simulink model "read_write_1"  (Simulink 7.9)
settings: Solver=ode45  StartTime=0.0  StopTime=50000  RelTol=1e-3
libraries: xbsIndex_r4 x71, xps_library x1
settings Model: Creator=peter  LastModifiedBy=peter

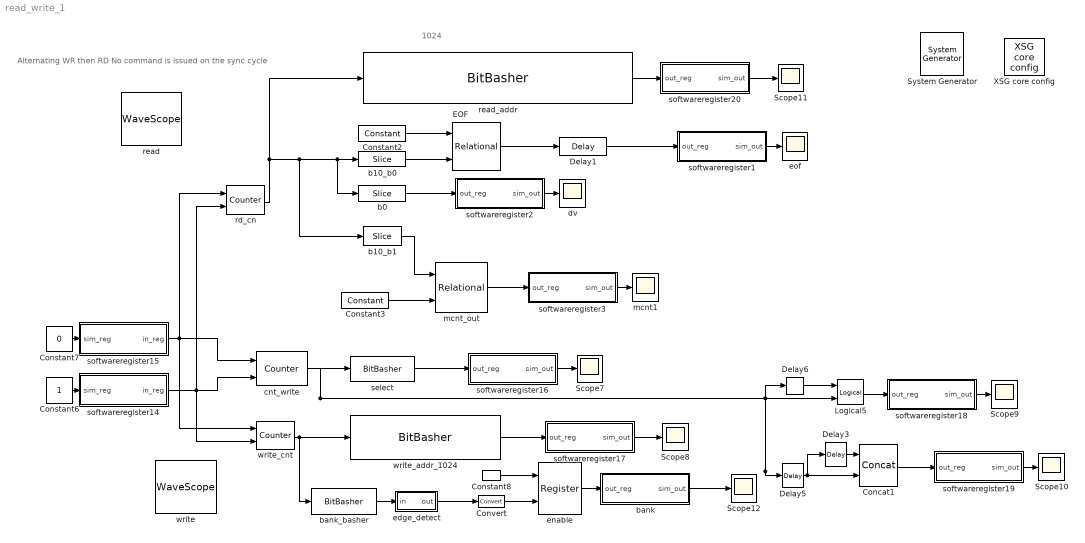
== system read_write_1 ==
  note: Alternating WR then RD
      | No command is issued
      | on the sync cycle
  note: 1024
  " System Generator" : xbsIndex_r4/ System Generator  Tag=genX  xilinxfamily=Kintex7  part=xc7k325t  speed=-3  package=fbg676  synthesis_tool=XST  clock_wrapper=Clock Enables  directory=./netlist  proj_type=Project Navigator  Synth_file=XST Defaults  Impl_file=ISE Defaults  testbench=off  simulink_period=1  sysclk_period=10  dcm_input_clock_period=10  incr_netlist=off  trim_vbits=Everywhere in SubSystem  dbl_ovrd=According to Block Masks  core_generation=According to Block Masks  run_coregen=off  deprecated_control=off  eval_field=0  block_type=sysgen
  Concat1 : xbsIndex_r4/Concat  num_inputs=2  dbl_ovrd=off  block_type=concat
      settings: block_version=10.1.3
  Constant2 : xbsIndex_r4/Constant  const=hex2dec('7FE')  gui_display_data_type=Fixed-point  arith_type=Unsigned  n_bits=11  bin_pt=0  preci_type=Single  exp_width=8  frac_width=24  explicit_period=on  period=1  equ=P=C  opselect=C  inp2=PCIN>>17  opr=+  inp1=P  carry=CIN  dbl_ovrd=off  block_type=constant
  Constant3 : xbsIndex_r4/Constant  const=hex2dec('7FE')  gui_display_data_type=Fixed-point  arith_type=Unsigned  n_bits=11  bin_pt=0  preci_type=Single  exp_width=8  frac_width=24  explicit_period=on  period=1  equ=P=C  opselect=C  inp2=PCIN>>17  opr=+  inp1=P  carry=CIN  dbl_ovrd=off  block_type=constant
  Constant6 : Constant
  Constant7 : Constant  Value=0
  Constant8 : xbsIndex_r4/Constant  const=1  gui_display_data_type=Boolean  arith_type=Boolean  n_bits=3  bin_pt=0  preci_type=Single  exp_width=8  frac_width=24  explicit_period=on  period=1  equ=P=C  opselect=C  inp2=PCIN>>17  opr=+  inp1=P  carry=CIN  dbl_ovrd=off  block_type=constant
  Convert : xbsIndex_r4/Convert  gui_display_data_type=Boolean  arith_type=Boolean  n_bits=16  bin_pt=14  float_type=Single  exp_bits=8  fraction_bits=24  quantization=Truncate  overflow=Wrap  en=off  latency=0  dbl_ovrd=off  pipeline=off  block_type=convert
  Delay1 : xbsIndex_r4/Delay  rst=off  infoeditControl=Selection of Reset will increase slice count due to use of real FFs and instead of SRLs  en=off  latency=1  dbl_ovrd=off  reg_retiming=off  block_type=delay
  Delay3 : xbsIndex_r4/Delay  rst=off  infoeditControl=Selection of Reset will increase slice count due to use of real FFs and instead of SRLs  en=off  latency=1  dbl_ovrd=off  reg_retiming=on  block_type=delay
      settings: xl_area=[0, 0, 0, 0, 0, 0, 0]
  Delay5 : xbsIndex_r4/Delay  rst=off  infoeditControl=Selection of Reset will increase slice count due to use of real FFs and instead of SRLs  en=off  latency=1  dbl_ovrd=off  reg_retiming=on  block_type=delay
      settings: xl_area=[0, 0, 0, 0, 0, 0, 0]
  Delay6 : xbsIndex_r4/Delay  rst=off  infoeditControl=Selection of Reset will increase slice count due to use of real FFs and instead of SRLs  en=off  latency=1  dbl_ovrd=off  reg_retiming=off  block_type=delay
      settings: xl_area=[0, 0, 0, 0, 0, 0, 0]
  EOF : xbsIndex_r4/Relational  mode=a=b  en=off  latency=1  dbl_ovrd=off  block_type=relational
  Logical5 : xbsIndex_r4/Logical  logical_function=XOR  inputs=2  en=off  latency=0  precision=Full  arith_type=Unsigned  n_bits=8  bin_pt=2  align_bp=on  dbl_ovrd=off  block_type=logical
      settings: xl_area=[0, 0, 0, 0, 0, 0, 0]
  Scope{7..12} (6 alike) : Scope
      Scope11 settings: ShowLegends=on  TimeRange=2500  YMin=0  YMax=8000  MaxDataPoints=1000000
      Scope12 settings: SaveName=ScopeData2
      Scope7 settings: YMin=-10  YMax=10  SaveName=ScopeData3
      Scope8 settings: ShowLegends=on  YMin=0  YMax=2050  SaveName=ScopeData4  MaxDataPoints=1000000
      Scope9 settings: SaveName=ScopeData5
  XSG core config : xps_library/XSG core config  Tag=xps:xsg  hw_sys=ROACH2:sx475t  clk_src=sys_clk  ROACH_clk_src=sys_clk  ROACH2_clk_src=sys_clk  clk_rate=100  sample_period=1  synthesis_tool=XST
  b0 : xbsIndex_r4/Slice  nbits=1  boolean_output=on  mode=Lower Bit Location + Width  bit1=0  base1=MSB of Input  bit0=0  base0=LSB of Input  dbl_ovrd=off  block_type=slice
  b10_b0 : xbsIndex_r4/Slice  nbits=11  boolean_output=off  mode=Lower Bit Location + Width  bit1=0  base1=MSB of Input  bit0=0  base0=LSB of Input  dbl_ovrd=off  block_type=slice
  b10_b1 : xbsIndex_r4/Slice  nbits=11  boolean_output=off  mode=Lower Bit Location + Width  bit1=0  base1=MSB of Input  bit0=0  base0=LSB of Input  dbl_ovrd=off  block_type=slice
  bank : Subsystem  Tag=xps:sw_reg  AncestorBlock=xps_library/software register  mask{numios=1, io_dir=To Processor, io_delay=0, sample_period=1, name1=reg, bitwidth1=1, arith_type1=Boolean, bin_pt1=0}
      mask prompts: numios "Num I/Os"; io_dir "I/O direction"; io_delay "I/O delay"; sample_period "Sample period"; name1 "Name"; bitwidth1 "Bitwidth"; arith_type1 "Type"; bin_pt1 "Binary pt"
      mask init:
      | swreg_init(gcb);
      mask StyleString: edit,popup(To Processor|From Processor),edit,edit,edit,edit,popup(Unsigned|Signed  (2's comp)|Boolean),edit
      mask CallbackString:
      | t = timer('StartDelay', 0.1); t.TimerFcn = {@swreg_cb, gcb}; start(t);|a = get_param(gcb, 'MaskEnables');
      | if strcmp(get_param(gcb, 'io_dir'), 'To Processor'),
      | a(4) = {'off'};
      | else
      | a(4) = {'on'};
      | end
      | set_param(gcb, 'MaskEnables', a);
      | |||||a = get_param(gcb, 'MaskEnables');
      | if strcmp(get_param(gcb, 'arith_type1'), 'Boolean'),
      | set_param(gcb, 'bitwidth1', '1');
      | set_param(gcb, 'bin_pt1', '0');
      | a(6) = {'off'};
      | a(8) = {'off'};
      | else
      | a(6) = {'on'};
      | a(8) = {'on'};
      | end
      | set_param(gcb, 'MaskEnables', a);
      | |
      mask TabNameString: Setup,Setup,Setup,Setup,IO1,IO1,IO1,IO1
  bank_basher : xbsIndex_r4/BitBasher  bitexpr=b={a[14]}  display_expr=on  sr_1=1  arith_type1=Unsigned  bin_pt1=0  sr_2=2  arith_type2=Unsigned  bin_pt2=0  sr_3=3  arith_type3=Unsigned  bin_pt3=0  sr_4=4  arith_type4=Unsigned  bin_pt4=0  dbl_ovrd=off  block_type=bitbasher
  cnt_write : xbsIndex_r4/Counter  cnt_type=Free Running  cnt_to=Inf  operation=Up  start_count=0  cnt_by_val=1  arith_type=Unsigned  n_bits=14  bin_pt=0  load_pin=off  rst=on  en=on  explicit_period=on  period=1  dbl_ovrd=off  use_behavioral_HDL=off  implementation=Fabric  use_rpm=off  block_type=counter
  dv : Scope
      settings: SaveName=ScopeData7
  edge_detect : Subsystem  AncestorBlock=casper_library_misc/edge_detect  mask(edge_detect){edge=Rising, polarity=Active High, x_in=[0 0.08 0.08 0.16 0.16 0.24 0.24 0.32 0.32 0.4], y_in=[-1 -1  1  1  1  1  1  1  1  1], x_out=[0.6 0.68 0.68 0.76 0.76 0.84 0.84 0.92 0.92 1], y_out=[-1 -1  1  1 -1 -1 -1 -1 -1 -1]}
      mask prompts: edge "Edge Type"; polarity "Output Polarity"; x_in "Input X Positions"; y_in "Input Y Positions"; x_out "Output X Positions"; y_out "Output Y Positions"
      mask help: Output is active for one-cycle after each edge of the specified type (i.e. rising, falling or both).
      mask init:
      | edge_detect_init(gcb,...
      |     'edge',edge,...
      |     'polarity',polarity,...
      |     'x_in',x_in,...
      |     'x_out',x_out,...
      |     'y_in',y_in,...
      |     'y_out',y_out);
      | 
      | x_in_num=str2num(getfield(getfield(get_param(gcb,'UserData'),'parameters'),'x_in'));
      | x_out_num=str2num(getfield(getfield(get_param(gcb,'UserData'),'parameters'),'x_out'));
      | y_in_num=str2num(getfield(getfield(get_param(gcb,'UserData'),'parameters'),'y_in'));
      | y_out_num=str2num(getfield(getfield(get_param(gcb,'UserData'),'parameters'),'y_out'));
      settings: AttributesFormatString=|
      | rising edges
      | active high
      mask Help: Output is active for one-cycle after each edge of the specified type (i.e. rising, falling, or both).  Latency is zero.
      mask StyleString: popup(Rising|Falling|Both),popup(Active High|Active Low),edit,edit,edit,edit
      mask Display:
      | plot(x_in_num,0.5+y_in_num*0.2);
      | plot(x_out_num,0.5+y_out_num*0.2);
  enable : xbsIndex_r4/Register  init=0  rst=off  en=on  dbl_ovrd=off  block_type=register
  eof : Scope
      settings: SaveName=ScopeData6
  mcnt1 : Scope
      settings: SaveName=ScopeData8
  mcnt_out : xbsIndex_r4/Relational  mode=a=b  en=off  latency=0  dbl_ovrd=off  block_type=relational
  rd_cn : xbsIndex_r4/Counter  cnt_type=Free Running  cnt_to=Inf  operation=Up  start_count=hex2dec('7FFE')  cnt_by_val=1  arith_type=Unsigned  n_bits=15  bin_pt=0  load_pin=off  rst=on  en=on  explicit_period=on  period=1  dbl_ovrd=off  use_behavioral_HDL=on  implementation=Fabric  use_rpm=off  block_type=counter
  read : xbsIndex_r4/WaveScope  block_type=wavescope
  read_addr : xbsIndex_r4/BitBasher  bitexpr=b={a[14],a[13:11],a[2],a[10:3],a[1]}  display_expr=on  sr_1=1  arith_type1=Unsigned  bin_pt1=0  sr_2=2  arith_type2=Unsigned  bin_pt2=0  sr_3=3  arith_type3=Unsigned  bin_pt3=0  sr_4=4  arith_type4=Unsigned  bin_pt4=0  dbl_ovrd=off  block_type=bitbasher
  select : xbsIndex_r4/BitBasher  bitexpr=b={a[8:7]}  display_expr=on  sr_1=1  arith_type1=Unsigned  bin_pt1=0  sr_2=2  arith_type2=Unsigned  bin_pt2=0  sr_3=3  arith_type3=Unsigned  bin_pt3=0  sr_4=4  arith_type4=Unsigned  bin_pt4=0  dbl_ovrd=off  block_type=bitbasher
  softwareregister1 : Subsystem  Tag=xps:sw_reg  AncestorBlock=xps_library/software register  mask{numios=1, io_dir=To Processor, io_delay=0, sample_period=1, name1=reg, bitwidth1=32, arith_type1=Unsigned, bin_pt1=0}
      mask prompts: numios "Num I/Os"; io_dir "I/O direction"; io_delay "I/O delay"; sample_period "Sample period"; name1 "Name"; bitwidth1 "Bitwidth"; arith_type1 "Type"; bin_pt1 "Binary pt"
      mask init:
      | swreg_init(gcb);
      mask StyleString: edit,popup(To Processor|From Processor),edit,edit,edit,edit,popup(Unsigned|Signed  (2's comp)|Boolean),edit
      mask CallbackString:
      | t = timer('StartDelay', 0.1); t.TimerFcn = {@swreg_cb, gcb}; start(t);|a = get_param(gcb, 'MaskEnables');
      | if strcmp(get_param(gcb, 'io_dir'), 'To Processor'),
      | a(4) = {'off'};
      | else
      | a(4) = {'on'};
      | end
      | set_param(gcb, 'MaskEnables', a);
      | |||||a = get_param(gcb, 'MaskEnables');
      | if strcmp(get_param(gcb, 'arith_type1'), 'Boolean'),
      | set_param(gcb, 'bitwidth1', '1');
      | set_param(gcb, 'bin_pt1', '0');
      | a(6) = {'off'};
      | a(8) = {'off'};
      | else
      | a(6) = {'on'};
      | a(8) = {'on'};
      | end
      | set_param(gcb, 'MaskEnables', a);
      | |
      mask TabNameString: Setup,Setup,Setup,Setup,IO1,IO1,IO1,IO1
  softwareregister14 : Subsystem  Tag=xps:sw_reg  AncestorBlock=xps_library/software register  mask{numios=1, io_dir=From Processor, io_delay=0, sample_period=1, name1=reg, bitwidth1=1, arith_type1=Boolean, bin_pt1=0}
      mask prompts: numios "Num I/Os"; io_dir "I/O direction"; io_delay "I/O delay"; sample_period "Sample period"; name1 "Name"; bitwidth1 "Bitwidth"; arith_type1 "Type"; bin_pt1 "Binary pt"
      mask init:
      | swreg_init(gcb);
      mask StyleString: edit,popup(To Processor|From Processor),edit,edit,edit,edit,popup(Unsigned|Signed  (2's comp)|Boolean),edit
      mask CallbackString:
      | t = timer('StartDelay', 0.1); t.TimerFcn = {@swreg_cb, gcb}; start(t);|a = get_param(gcb, 'MaskEnables');
      | if strcmp(get_param(gcb, 'io_dir'), 'To Processor'),
      | a(4) = {'off'};
      | else
      | a(4) = {'on'};
      | end
      | set_param(gcb, 'MaskEnables', a);
      | |||||a = get_param(gcb, 'MaskEnables');
      | if strcmp(get_param(gcb, 'arith_type1'), 'Boolean'),
      | set_param(gcb, 'bitwidth1', '1');
      | set_param(gcb, 'bin_pt1', '0');
      | a(6) = {'off'};
      | a(8) = {'off'};
      | else
      | a(6) = {'on'};
      | a(8) = {'on'};
      | end
      | set_param(gcb, 'MaskEnables', a);
      | |
      mask TabNameString: Setup,Setup,Setup,Setup,IO1,IO1,IO1,IO1
  softwareregister15 : Subsystem  Tag=xps:sw_reg  AncestorBlock=xps_library/software register  mask{numios=1, io_dir=From Processor, io_delay=0, sample_period=1, name1=reg, bitwidth1=1, arith_type1=Boolean, bin_pt1=0}
      mask prompts: numios "Num I/Os"; io_dir "I/O direction"; io_delay "I/O delay"; sample_period "Sample period"; name1 "Name"; bitwidth1 "Bitwidth"; arith_type1 "Type"; bin_pt1 "Binary pt"
      mask init:
      | swreg_init(gcb);
      mask StyleString: edit,popup(To Processor|From Processor),edit,edit,edit,edit,popup(Unsigned|Signed  (2's comp)|Boolean),edit
      mask CallbackString:
      | t = timer('StartDelay', 0.1); t.TimerFcn = {@swreg_cb, gcb}; start(t);|a = get_param(gcb, 'MaskEnables');
      | if strcmp(get_param(gcb, 'io_dir'), 'To Processor'),
      | a(4) = {'off'};
      | else
      | a(4) = {'on'};
      | end
      | set_param(gcb, 'MaskEnables', a);
      | |||||a = get_param(gcb, 'MaskEnables');
      | if strcmp(get_param(gcb, 'arith_type1'), 'Boolean'),
      | set_param(gcb, 'bitwidth1', '1');
      | set_param(gcb, 'bin_pt1', '0');
      | a(6) = {'off'};
      | a(8) = {'off'};
      | else
      | a(6) = {'on'};
      | a(8) = {'on'};
      | end
      | set_param(gcb, 'MaskEnables', a);
      | |
      mask TabNameString: Setup,Setup,Setup,Setup,IO1,IO1,IO1,IO1
  softwareregister16 : Subsystem  Tag=xps:sw_reg  AncestorBlock=xps_library/software register  mask{numios=1, io_dir=To Processor, io_delay=0, sample_period=1, name1=reg, bitwidth1=32, arith_type1=Unsigned, bin_pt1=0}
      mask prompts: numios "Num I/Os"; io_dir "I/O direction"; io_delay "I/O delay"; sample_period "Sample period"; name1 "Name"; bitwidth1 "Bitwidth"; arith_type1 "Type"; bin_pt1 "Binary pt"
      mask init:
      | swreg_init(gcb);
      mask StyleString: edit,popup(To Processor|From Processor),edit,edit,edit,edit,popup(Unsigned|Signed  (2's comp)|Boolean),edit
      mask CallbackString:
      | t = timer('StartDelay', 0.1); t.TimerFcn = {@swreg_cb, gcb}; start(t);|a = get_param(gcb, 'MaskEnables');
      | if strcmp(get_param(gcb, 'io_dir'), 'To Processor'),
      | a(4) = {'off'};
      | else
      | a(4) = {'on'};
      | end
      | set_param(gcb, 'MaskEnables', a);
      | |||||a = get_param(gcb, 'MaskEnables');
      | if strcmp(get_param(gcb, 'arith_type1'), 'Boolean'),
      | set_param(gcb, 'bitwidth1', '1');
      | set_param(gcb, 'bin_pt1', '0');
      | a(6) = {'off'};
      | a(8) = {'off'};
      | else
      | a(6) = {'on'};
      | a(8) = {'on'};
      | end
      | set_param(gcb, 'MaskEnables', a);
      | |
      mask TabNameString: Setup,Setup,Setup,Setup,IO1,IO1,IO1,IO1
  softwareregister17 : Subsystem  Tag=xps:sw_reg  AncestorBlock=xps_library/software register  mask{numios=1, io_dir=To Processor, io_delay=0, sample_period=1, name1=reg, bitwidth1=14, arith_type1=Unsigned, bin_pt1=0}
      mask prompts: numios "Num I/Os"; io_dir "I/O direction"; io_delay "I/O delay"; sample_period "Sample period"; name1 "Name"; bitwidth1 "Bitwidth"; arith_type1 "Type"; bin_pt1 "Binary pt"
      mask init:
      | swreg_init(gcb);
      mask StyleString: edit,popup(To Processor|From Processor),edit,edit,edit,edit,popup(Unsigned|Signed  (2's comp)|Boolean),edit
      mask CallbackString:
      | t = timer('StartDelay', 0.1); t.TimerFcn = {@swreg_cb, gcb}; start(t);|a = get_param(gcb, 'MaskEnables');
      | if strcmp(get_param(gcb, 'io_dir'), 'To Processor'),
      | a(4) = {'off'};
      | else
      | a(4) = {'on'};
      | end
      | set_param(gcb, 'MaskEnables', a);
      | |||||a = get_param(gcb, 'MaskEnables');
      | if strcmp(get_param(gcb, 'arith_type1'), 'Boolean'),
      | set_param(gcb, 'bitwidth1', '1');
      | set_param(gcb, 'bin_pt1', '0');
      | a(6) = {'off'};
      | a(8) = {'off'};
      | else
      | a(6) = {'on'};
      | a(8) = {'on'};
      | end
      | set_param(gcb, 'MaskEnables', a);
      | |
      mask TabNameString: Setup,Setup,Setup,Setup,IO1,IO1,IO1,IO1
  softwareregister18 : Subsystem  Tag=xps:sw_reg  AncestorBlock=xps_library/software register  mask{numios=1, io_dir=To Processor, io_delay=0, sample_period=1, name1=reg, bitwidth1=32, arith_type1=Unsigned, bin_pt1=0}
      mask prompts: numios "Num I/Os"; io_dir "I/O direction"; io_delay "I/O delay"; sample_period "Sample period"; name1 "Name"; bitwidth1 "Bitwidth"; arith_type1 "Type"; bin_pt1 "Binary pt"
      mask init:
      | swreg_init(gcb);
      mask StyleString: edit,popup(To Processor|From Processor),edit,edit,edit,edit,popup(Unsigned|Signed  (2's comp)|Boolean),edit
      mask CallbackString:
      | t = timer('StartDelay', 0.1); t.TimerFcn = {@swreg_cb, gcb}; start(t);|a = get_param(gcb, 'MaskEnables');
      | if strcmp(get_param(gcb, 'io_dir'), 'To Processor'),
      | a(4) = {'off'};
      | else
      | a(4) = {'on'};
      | end
      | set_param(gcb, 'MaskEnables', a);
      | |||||a = get_param(gcb, 'MaskEnables');
      | if strcmp(get_param(gcb, 'arith_type1'), 'Boolean'),
      | set_param(gcb, 'bitwidth1', '1');
      | set_param(gcb, 'bin_pt1', '0');
      | a(6) = {'off'};
      | a(8) = {'off'};
      | else
      | a(6) = {'on'};
      | a(8) = {'on'};
      | end
      | set_param(gcb, 'MaskEnables', a);
      | |
      mask TabNameString: Setup,Setup,Setup,Setup,IO1,IO1,IO1,IO1
  softwareregister19 : Subsystem  Tag=xps:sw_reg  AncestorBlock=xps_library/software register  mask{numios=1, io_dir=To Processor, io_delay=0, sample_period=1, name1=reg, bitwidth1=32, arith_type1=Unsigned, bin_pt1=0}
      mask prompts: numios "Num I/Os"; io_dir "I/O direction"; io_delay "I/O delay"; sample_period "Sample period"; name1 "Name"; bitwidth1 "Bitwidth"; arith_type1 "Type"; bin_pt1 "Binary pt"
      mask init:
      | swreg_init(gcb);
      mask StyleString: edit,popup(To Processor|From Processor),edit,edit,edit,edit,popup(Unsigned|Signed  (2's comp)|Boolean),edit
      mask CallbackString:
      | t = timer('StartDelay', 0.1); t.TimerFcn = {@swreg_cb, gcb}; start(t);|a = get_param(gcb, 'MaskEnables');
      | if strcmp(get_param(gcb, 'io_dir'), 'To Processor'),
      | a(4) = {'off'};
      | else
      | a(4) = {'on'};
      | end
      | set_param(gcb, 'MaskEnables', a);
      | |||||a = get_param(gcb, 'MaskEnables');
      | if strcmp(get_param(gcb, 'arith_type1'), 'Boolean'),
      | set_param(gcb, 'bitwidth1', '1');
      | set_param(gcb, 'bin_pt1', '0');
      | a(6) = {'off'};
      | a(8) = {'off'};
      | else
      | a(6) = {'on'};
      | a(8) = {'on'};
      | end
      | set_param(gcb, 'MaskEnables', a);
      | |
      mask TabNameString: Setup,Setup,Setup,Setup,IO1,IO1,IO1,IO1
  softwareregister2 : Subsystem  Tag=xps:sw_reg  AncestorBlock=xps_library/software register  mask{numios=1, io_dir=To Processor, io_delay=0, sample_period=1, name1=reg, bitwidth1=32, arith_type1=Unsigned, bin_pt1=0}
      mask prompts: numios "Num I/Os"; io_dir "I/O direction"; io_delay "I/O delay"; sample_period "Sample period"; name1 "Name"; bitwidth1 "Bitwidth"; arith_type1 "Type"; bin_pt1 "Binary pt"
      mask init:
      | swreg_init(gcb);
      mask StyleString: edit,popup(To Processor|From Processor),edit,edit,edit,edit,popup(Unsigned|Signed  (2's comp)|Boolean),edit
      mask CallbackString:
      | t = timer('StartDelay', 0.1); t.TimerFcn = {@swreg_cb, gcb}; start(t);|a = get_param(gcb, 'MaskEnables');
      | if strcmp(get_param(gcb, 'io_dir'), 'To Processor'),
      | a(4) = {'off'};
      | else
      | a(4) = {'on'};
      | end
      | set_param(gcb, 'MaskEnables', a);
      | |||||a = get_param(gcb, 'MaskEnables');
      | if strcmp(get_param(gcb, 'arith_type1'), 'Boolean'),
      | set_param(gcb, 'bitwidth1', '1');
      | set_param(gcb, 'bin_pt1', '0');
      | a(6) = {'off'};
      | a(8) = {'off'};
      | else
      | a(6) = {'on'};
      | a(8) = {'on'};
      | end
      | set_param(gcb, 'MaskEnables', a);
      | |
      mask TabNameString: Setup,Setup,Setup,Setup,IO1,IO1,IO1,IO1
  softwareregister20 : Subsystem  Tag=xps:sw_reg  AncestorBlock=xps_library/software register  mask{numios=1, io_dir=To Processor, io_delay=0, sample_period=1, name1=reg, bitwidth1=15, arith_type1=Unsigned, bin_pt1=0}
      mask prompts: numios "Num I/Os"; io_dir "I/O direction"; io_delay "I/O delay"; sample_period "Sample period"; name1 "Name"; bitwidth1 "Bitwidth"; arith_type1 "Type"; bin_pt1 "Binary pt"
      mask init:
      | swreg_init(gcb);
      mask StyleString: edit,popup(To Processor|From Processor),edit,edit,edit,edit,popup(Unsigned|Signed  (2's comp)|Boolean),edit
      mask CallbackString:
      | t = timer('StartDelay', 0.1); t.TimerFcn = {@swreg_cb, gcb}; start(t);|a = get_param(gcb, 'MaskEnables');
      | if strcmp(get_param(gcb, 'io_dir'), 'To Processor'),
      | a(4) = {'off'};
      | else
      | a(4) = {'on'};
      | end
      | set_param(gcb, 'MaskEnables', a);
      | |||||a = get_param(gcb, 'MaskEnables');
      | if strcmp(get_param(gcb, 'arith_type1'), 'Boolean'),
      | set_param(gcb, 'bitwidth1', '1');
      | set_param(gcb, 'bin_pt1', '0');
      | a(6) = {'off'};
      | a(8) = {'off'};
      | else
      | a(6) = {'on'};
      | a(8) = {'on'};
      | end
      | set_param(gcb, 'MaskEnables', a);
      | |
      mask TabNameString: Setup,Setup,Setup,Setup,IO1,IO1,IO1,IO1
  softwareregister3 : Subsystem  Tag=xps:sw_reg  AncestorBlock=xps_library/software register  mask{numios=1, io_dir=To Processor, io_delay=0, sample_period=1, name1=reg, bitwidth1=32, arith_type1=Unsigned, bin_pt1=0}
      mask prompts: numios "Num I/Os"; io_dir "I/O direction"; io_delay "I/O delay"; sample_period "Sample period"; name1 "Name"; bitwidth1 "Bitwidth"; arith_type1 "Type"; bin_pt1 "Binary pt"
      mask init:
      | swreg_init(gcb);
      mask StyleString: edit,popup(To Processor|From Processor),edit,edit,edit,edit,popup(Unsigned|Signed  (2's comp)|Boolean),edit
      mask CallbackString:
      | t = timer('StartDelay', 0.1); t.TimerFcn = {@swreg_cb, gcb}; start(t);|a = get_param(gcb, 'MaskEnables');
      | if strcmp(get_param(gcb, 'io_dir'), 'To Processor'),
      | a(4) = {'off'};
      | else
      | a(4) = {'on'};
      | end
      | set_param(gcb, 'MaskEnables', a);
      | |||||a = get_param(gcb, 'MaskEnables');
      | if strcmp(get_param(gcb, 'arith_type1'), 'Boolean'),
      | set_param(gcb, 'bitwidth1', '1');
      | set_param(gcb, 'bin_pt1', '0');
      | a(6) = {'off'};
      | a(8) = {'off'};
      | else
      | a(6) = {'on'};
      | a(8) = {'on'};
      | end
      | set_param(gcb, 'MaskEnables', a);
      | |
      mask TabNameString: Setup,Setup,Setup,Setup,IO1,IO1,IO1,IO1
  write : xbsIndex_r4/WaveScope  block_type=wavescope
  write_addr_1024 : xbsIndex_r4/BitBasher  bitexpr=b={a[14:10],a[7:0]}  display_expr=on  sr_1=1  arith_type1=Unsigned  bin_pt1=0  sr_2=2  arith_type2=Unsigned  bin_pt2=0  sr_3=3  arith_type3=Unsigned  bin_pt3=0  sr_4=4  arith_type4=Unsigned  bin_pt4=0  dbl_ovrd=off  block_type=bitbasher
  write_cnt : xbsIndex_r4/Counter  cnt_type=Free Running  cnt_to=Inf  operation=Up  start_count=0  cnt_by_val=1  arith_type=Unsigned  n_bits=15  bin_pt=0  load_pin=off  rst=on  en=on  explicit_period=on  period=1  dbl_ovrd=off  use_behavioral_HDL=off  implementation=Fabric  use_rpm=off  block_type=counter
  wires:
  Constant6/1 -> softwareregister14/1(sim_reg)
  Constant7/1 -> softwareregister15/1(sim_reg)
  softwareregister15/1(in_reg) -> cnt_write/1, write_cnt/1, rd_cn/1
  softwareregister14/1(in_reg) -> cnt_write/2, write_cnt/2, rd_cn/2
  cnt_write/1 -> Delay6/1, Logical5/2, Delay5/1, select/1
  softwareregister16/1(sim_out) -> Scope7/1
  write_cnt/1 -> write_addr_1024/1, bank_basher/1
  softwareregister17/1(sim_out) -> Scope8/1
  write_addr_1024/1 -> softwareregister17/1(out_reg)
  Delay6/1 -> Logical5/1
  Logical5/1 -> softwareregister18/1(out_reg)
  softwareregister18/1(sim_out) -> Scope9/1
  Delay3/1 -> Concat1/1
  Delay5/1 -> Concat1/2, Delay3/1
  softwareregister19/1(sim_out) -> Scope10/1
  Concat1/1 -> softwareregister19/1(out_reg)
  softwareregister20/1(sim_out) -> Scope11/1
  read_addr/1 -> softwareregister20/1(out_reg)
  rd_cn/1 -> read_addr/1, b10_b0/1, b0/1, b10_b1/1
  select/1 -> softwareregister16/1(out_reg)
  bank/1(sim_out) -> Scope12/1
  bank_basher/1 -> edge_detect/1(in)
  Constant8/1 -> enable/1
  edge_detect/1(out) -> Convert/1
  enable/1 -> bank/1(out_reg)
  Convert/1 -> enable/2
  Constant2/1 -> EOF/1
  b10_b0/1 -> EOF/2
  EOF/1 -> Delay1/1
  softwareregister1/1(sim_out) -> eof/1
  Delay1/1 -> softwareregister1/1(out_reg)
  softwareregister2/1(sim_out) -> dv/1
  b0/1 -> softwareregister2/1(out_reg)
  softwareregister3/1(sim_out) -> mcnt1/1
  Constant3/1 -> mcnt_out/2
  mcnt_out/1 -> softwareregister3/1(out_reg)
  b10_b1/1 -> mcnt_out/1

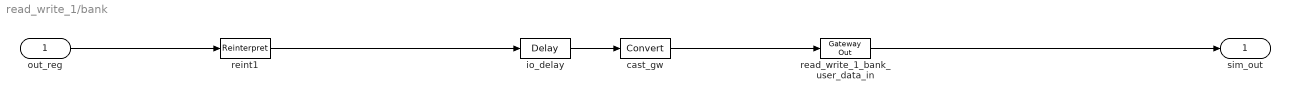
== system read_write_1/bank ==
  out_reg : Inport
  cast_gw : xbsIndex_r4/Convert  gui_display_data_type=Fixed-point  arith_type=Unsigned  n_bits=32  bin_pt=0  float_type=Single  exp_bits=8  fraction_bits=24  quantization=Truncate  overflow=Wrap  en=off  latency=0  dbl_ovrd=off  pipeline=off  block_type=convert
  io_delay : xbsIndex_r4/Delay  rst=off  infoeditControl=Selection of Reset will increase slice count due to use of real FFs and instead of SRLs  en=off  latency=0  dbl_ovrd=off  reg_retiming=on  block_type=delay
  read_write_1_bank_user_data_in : xbsIndex_r4/Gateway Out  inherit_from_input=off  hdl_port=on  timing_constraint=None  locs_specified=off  LOCs={}  UseAsDAC=off  DACChannel='1'  block_type=gatewayout
  reint1 : xbsIndex_r4/Reinterpret  force_arith_type=on  arith_type=Unsigned  force_bin_pt=on  bin_pt=0  block_type=reinterpret
  sim_out : Outport
  wires:
  io_delay/1 -> cast_gw/1
  cast_gw/1 -> read_write_1_bank_user_data_in/1
  read_write_1_bank_user_data_in/1 -> sim_out/1
  out_reg/1 -> reint1/1
  reint1/1 -> io_delay/1

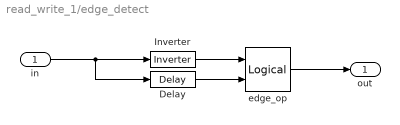
== system read_write_1/edge_detect ==
  in : Inport
  Delay : xbsIndex_r4/Delay  rst=off  infoeditControl=Selection of Reset will increase slice count due to use of real FFs and instead of SRLs  en=off  latency=1  dbl_ovrd=off  reg_retiming=off  block_type=delay
      settings: xl_area=[0, 0, 0, 0, 0, 0, 0]
  Inverter : xbsIndex_r4/Inverter  en=off  latency=0  dbl_ovrd=off  block_type=inv
      settings: xl_area=[0, 0, 0, 0, 0, 0, 0]
  edge_op : xbsIndex_r4/Logical  logical_function=NOR  inputs=2  en=off  latency=0  precision=Full  arith_type=Unsigned  n_bits=8  bin_pt=2  align_bp=on  dbl_ovrd=off  block_type=logical
      settings: xl_area=[0, 0, 0, 0, 0, 0, 0]
  out : Outport
  wires:
  Inverter/1 -> edge_op/1
  edge_op/1 -> out/1
  in/1 -> Inverter/1, Delay/1
  Delay/1 -> edge_op/2

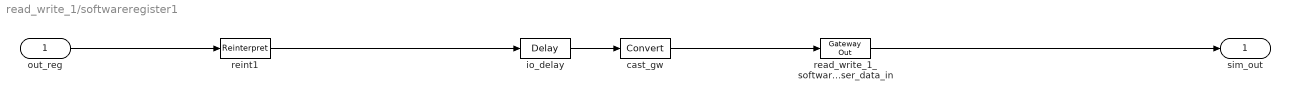
== system read_write_1/softwareregister1 ==
  out_reg : Inport
  cast_gw : xbsIndex_r4/Convert  gui_display_data_type=Fixed-point  arith_type=Unsigned  n_bits=32  bin_pt=0  float_type=Single  exp_bits=8  fraction_bits=24  quantization=Truncate  overflow=Wrap  en=off  latency=0  dbl_ovrd=off  pipeline=off  block_type=convert
  io_delay : xbsIndex_r4/Delay  rst=off  infoeditControl=Selection of Reset will increase slice count due to use of real FFs and instead of SRLs  en=off  latency=0  dbl_ovrd=off  reg_retiming=on  block_type=delay
  read_write_1_softwareregister1_user_data_in : xbsIndex_r4/Gateway Out  inherit_from_input=off  hdl_port=on  timing_constraint=None  locs_specified=off  LOCs={}  UseAsDAC=off  DACChannel='1'  block_type=gatewayout
  reint1 : xbsIndex_r4/Reinterpret  force_arith_type=on  arith_type=Unsigned  force_bin_pt=on  bin_pt=0  block_type=reinterpret
  sim_out : Outport
  wires:
  io_delay/1 -> cast_gw/1
  cast_gw/1 -> read_write_1_softwareregister1_user_data_in/1
  read_write_1_softwareregister1_user_data_in/1 -> sim_out/1
  out_reg/1 -> reint1/1
  reint1/1 -> io_delay/1

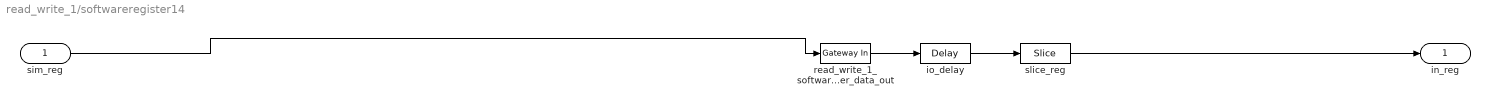
== system read_write_1/softwareregister14 ==
  sim_reg : Inport
  io_delay : xbsIndex_r4/Delay  rst=off  infoeditControl=Selection of Reset will increase slice count due to use of real FFs and instead of SRLs  en=off  latency=0  dbl_ovrd=off  reg_retiming=on  block_type=delay
  read_write_1_softwareregister14_user_data_out : xbsIndex_r4/Gateway In  gui_display_data_type=Fixed-point  arith_type=Unsigned  n_bits=32  bin_pt=0  preci_type=Single  exp_width=8  frac_width=24  quantization="Round  (unbiased: +/- Inf)"  overflow=Saturate  period=1  dbl_ovrd=off  timing_constraint=None  locs_specified=off  LOCs={}  UseAsADC=off  ADCChannel='1'  inherit_from_input=off  hdl_port=on  block_type=gatewayin
  slice_reg : xbsIndex_r4/Slice  nbits=1  boolean_output=on  mode=Lower Bit Location + Width  bit1=0  base1=MSB of Input  bit0=0  base0=LSB of Input  dbl_ovrd=off  block_type=slice
  in_reg : Outport
  wires:
  read_write_1_softwareregister14_user_data_out/1 -> io_delay/1
  sim_reg/1 -> read_write_1_softwareregister14_user_data_out/1
  io_delay/1 -> slice_reg/1
  slice_reg/1 -> in_reg/1

== system read_write_1/softwareregister15 ==
  sim_reg : Inport
  io_delay : xbsIndex_r4/Delay  rst=off  infoeditControl=Selection of Reset will increase slice count due to use of real FFs and instead of SRLs  en=off  latency=0  dbl_ovrd=off  reg_retiming=on  block_type=delay
  read_write_1_softwareregister15_user_data_out : xbsIndex_r4/Gateway In  gui_display_data_type=Fixed-point  arith_type=Unsigned  n_bits=32  bin_pt=0  preci_type=Single  exp_width=8  frac_width=24  quantization="Round  (unbiased: +/- Inf)"  overflow=Saturate  period=1  dbl_ovrd=off  timing_constraint=None  locs_specified=off  LOCs={}  UseAsADC=off  ADCChannel='1'  inherit_from_input=off  hdl_port=on  block_type=gatewayin
  slice_reg : xbsIndex_r4/Slice  nbits=1  boolean_output=on  mode=Lower Bit Location + Width  bit1=0  base1=MSB of Input  bit0=0  base0=LSB of Input  dbl_ovrd=off  block_type=slice
  in_reg : Outport
  wires:
  read_write_1_softwareregister15_user_data_out/1 -> io_delay/1
  sim_reg/1 -> read_write_1_softwareregister15_user_data_out/1
  io_delay/1 -> slice_reg/1
  slice_reg/1 -> in_reg/1

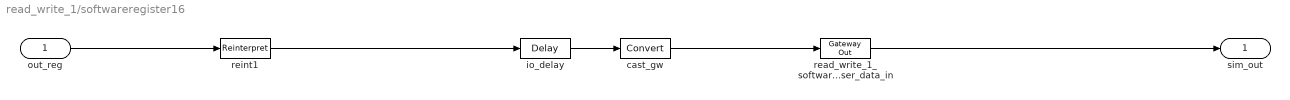
== system read_write_1/softwareregister16 ==
  out_reg : Inport
  cast_gw : xbsIndex_r4/Convert  gui_display_data_type=Fixed-point  arith_type=Unsigned  n_bits=32  bin_pt=0  float_type=Single  exp_bits=8  fraction_bits=24  quantization=Truncate  overflow=Wrap  en=off  latency=0  dbl_ovrd=off  pipeline=off  block_type=convert
  io_delay : xbsIndex_r4/Delay  rst=off  infoeditControl=Selection of Reset will increase slice count due to use of real FFs and instead of SRLs  en=off  latency=0  dbl_ovrd=off  reg_retiming=on  block_type=delay
  read_write_1_softwareregister16_user_data_in : xbsIndex_r4/Gateway Out  inherit_from_input=off  hdl_port=on  timing_constraint=None  locs_specified=off  LOCs={}  UseAsDAC=off  DACChannel='1'  block_type=gatewayout
  reint1 : xbsIndex_r4/Reinterpret  force_arith_type=on  arith_type=Unsigned  force_bin_pt=on  bin_pt=0  block_type=reinterpret
  sim_out : Outport
  wires:
  io_delay/1 -> cast_gw/1
  cast_gw/1 -> read_write_1_softwareregister16_user_data_in/1
  read_write_1_softwareregister16_user_data_in/1 -> sim_out/1
  out_reg/1 -> reint1/1
  reint1/1 -> io_delay/1

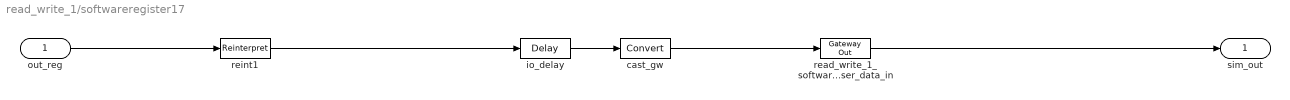
== system read_write_1/softwareregister17 ==
  out_reg : Inport
  cast_gw : xbsIndex_r4/Convert  gui_display_data_type=Fixed-point  arith_type=Unsigned  n_bits=32  bin_pt=0  float_type=Single  exp_bits=8  fraction_bits=24  quantization=Truncate  overflow=Wrap  en=off  latency=0  dbl_ovrd=off  pipeline=off  block_type=convert
  io_delay : xbsIndex_r4/Delay  rst=off  infoeditControl=Selection of Reset will increase slice count due to use of real FFs and instead of SRLs  en=off  latency=0  dbl_ovrd=off  reg_retiming=on  block_type=delay
  read_write_1_softwareregister17_user_data_in : xbsIndex_r4/Gateway Out  inherit_from_input=off  hdl_port=on  timing_constraint=None  locs_specified=off  LOCs={}  UseAsDAC=off  DACChannel='1'  block_type=gatewayout
  reint1 : xbsIndex_r4/Reinterpret  force_arith_type=on  arith_type=Unsigned  force_bin_pt=on  bin_pt=0  block_type=reinterpret
  sim_out : Outport
  wires:
  io_delay/1 -> cast_gw/1
  cast_gw/1 -> read_write_1_softwareregister17_user_data_in/1
  read_write_1_softwareregister17_user_data_in/1 -> sim_out/1
  out_reg/1 -> reint1/1
  reint1/1 -> io_delay/1

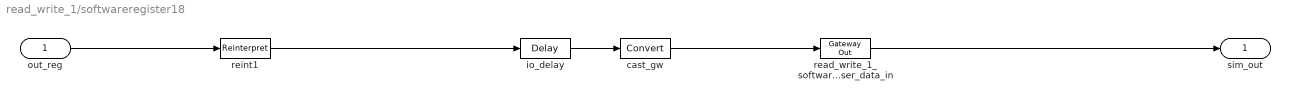
== system read_write_1/softwareregister18 ==
  out_reg : Inport
  cast_gw : xbsIndex_r4/Convert  gui_display_data_type=Fixed-point  arith_type=Unsigned  n_bits=32  bin_pt=0  float_type=Single  exp_bits=8  fraction_bits=24  quantization=Truncate  overflow=Wrap  en=off  latency=0  dbl_ovrd=off  pipeline=off  block_type=convert
  io_delay : xbsIndex_r4/Delay  rst=off  infoeditControl=Selection of Reset will increase slice count due to use of real FFs and instead of SRLs  en=off  latency=0  dbl_ovrd=off  reg_retiming=on  block_type=delay
  read_write_1_softwareregister18_user_data_in : xbsIndex_r4/Gateway Out  inherit_from_input=off  hdl_port=on  timing_constraint=None  locs_specified=off  LOCs={}  UseAsDAC=off  DACChannel='1'  block_type=gatewayout
  reint1 : xbsIndex_r4/Reinterpret  force_arith_type=on  arith_type=Unsigned  force_bin_pt=on  bin_pt=0  block_type=reinterpret
  sim_out : Outport
  wires:
  io_delay/1 -> cast_gw/1
  cast_gw/1 -> read_write_1_softwareregister18_user_data_in/1
  read_write_1_softwareregister18_user_data_in/1 -> sim_out/1
  out_reg/1 -> reint1/1
  reint1/1 -> io_delay/1

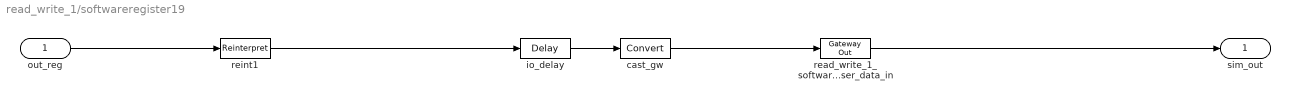
== system read_write_1/softwareregister19 ==
  out_reg : Inport
  cast_gw : xbsIndex_r4/Convert  gui_display_data_type=Fixed-point  arith_type=Unsigned  n_bits=32  bin_pt=0  float_type=Single  exp_bits=8  fraction_bits=24  quantization=Truncate  overflow=Wrap  en=off  latency=0  dbl_ovrd=off  pipeline=off  block_type=convert
  io_delay : xbsIndex_r4/Delay  rst=off  infoeditControl=Selection of Reset will increase slice count due to use of real FFs and instead of SRLs  en=off  latency=0  dbl_ovrd=off  reg_retiming=on  block_type=delay
  read_write_1_softwareregister19_user_data_in : xbsIndex_r4/Gateway Out  inherit_from_input=off  hdl_port=on  timing_constraint=None  locs_specified=off  LOCs={}  UseAsDAC=off  DACChannel='1'  block_type=gatewayout
  reint1 : xbsIndex_r4/Reinterpret  force_arith_type=on  arith_type=Unsigned  force_bin_pt=on  bin_pt=0  block_type=reinterpret
  sim_out : Outport
  wires:
  io_delay/1 -> cast_gw/1
  cast_gw/1 -> read_write_1_softwareregister19_user_data_in/1
  read_write_1_softwareregister19_user_data_in/1 -> sim_out/1
  out_reg/1 -> reint1/1
  reint1/1 -> io_delay/1

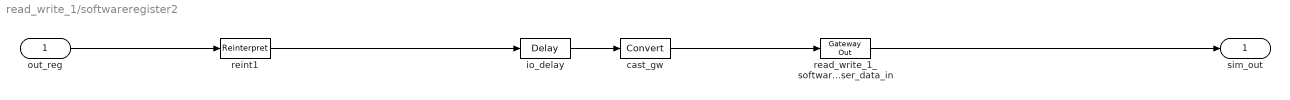
== system read_write_1/softwareregister2 ==
  out_reg : Inport
  cast_gw : xbsIndex_r4/Convert  gui_display_data_type=Fixed-point  arith_type=Unsigned  n_bits=32  bin_pt=0  float_type=Single  exp_bits=8  fraction_bits=24  quantization=Truncate  overflow=Wrap  en=off  latency=0  dbl_ovrd=off  pipeline=off  block_type=convert
  io_delay : xbsIndex_r4/Delay  rst=off  infoeditControl=Selection of Reset will increase slice count due to use of real FFs and instead of SRLs  en=off  latency=0  dbl_ovrd=off  reg_retiming=on  block_type=delay
  read_write_1_softwareregister2_user_data_in : xbsIndex_r4/Gateway Out  inherit_from_input=off  hdl_port=on  timing_constraint=None  locs_specified=off  LOCs={}  UseAsDAC=off  DACChannel='1'  block_type=gatewayout
  reint1 : xbsIndex_r4/Reinterpret  force_arith_type=on  arith_type=Unsigned  force_bin_pt=on  bin_pt=0  block_type=reinterpret
  sim_out : Outport
  wires:
  io_delay/1 -> cast_gw/1
  cast_gw/1 -> read_write_1_softwareregister2_user_data_in/1
  read_write_1_softwareregister2_user_data_in/1 -> sim_out/1
  out_reg/1 -> reint1/1
  reint1/1 -> io_delay/1

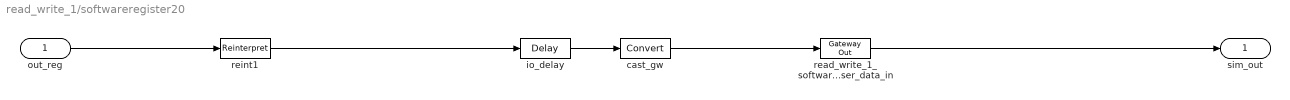
== system read_write_1/softwareregister20 ==
  out_reg : Inport
  cast_gw : xbsIndex_r4/Convert  gui_display_data_type=Fixed-point  arith_type=Unsigned  n_bits=32  bin_pt=0  float_type=Single  exp_bits=8  fraction_bits=24  quantization=Truncate  overflow=Wrap  en=off  latency=0  dbl_ovrd=off  pipeline=off  block_type=convert
  io_delay : xbsIndex_r4/Delay  rst=off  infoeditControl=Selection of Reset will increase slice count due to use of real FFs and instead of SRLs  en=off  latency=0  dbl_ovrd=off  reg_retiming=on  block_type=delay
  read_write_1_softwareregister20_user_data_in : xbsIndex_r4/Gateway Out  inherit_from_input=off  hdl_port=on  timing_constraint=None  locs_specified=off  LOCs={}  UseAsDAC=off  DACChannel='1'  block_type=gatewayout
  reint1 : xbsIndex_r4/Reinterpret  force_arith_type=on  arith_type=Unsigned  force_bin_pt=on  bin_pt=0  block_type=reinterpret
  sim_out : Outport
  wires:
  io_delay/1 -> cast_gw/1
  cast_gw/1 -> read_write_1_softwareregister20_user_data_in/1
  read_write_1_softwareregister20_user_data_in/1 -> sim_out/1
  out_reg/1 -> reint1/1
  reint1/1 -> io_delay/1

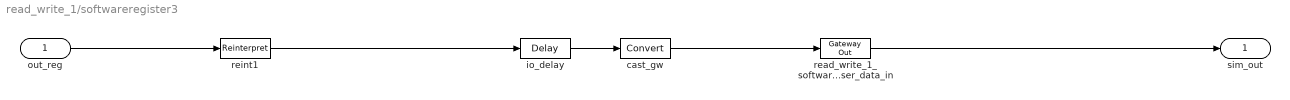
== system read_write_1/softwareregister3 ==
  out_reg : Inport
  cast_gw : xbsIndex_r4/Convert  gui_display_data_type=Fixed-point  arith_type=Unsigned  n_bits=32  bin_pt=0  float_type=Single  exp_bits=8  fraction_bits=24  quantization=Truncate  overflow=Wrap  en=off  latency=0  dbl_ovrd=off  pipeline=off  block_type=convert
  io_delay : xbsIndex_r4/Delay  rst=off  infoeditControl=Selection of Reset will increase slice count due to use of real FFs and instead of SRLs  en=off  latency=0  dbl_ovrd=off  reg_retiming=on  block_type=delay
  read_write_1_softwareregister3_user_data_in : xbsIndex_r4/Gateway Out  inherit_from_input=off  hdl_port=on  timing_constraint=None  locs_specified=off  LOCs={}  UseAsDAC=off  DACChannel='1'  block_type=gatewayout
  reint1 : xbsIndex_r4/Reinterpret  force_arith_type=on  arith_type=Unsigned  force_bin_pt=on  bin_pt=0  block_type=reinterpret
  sim_out : Outport
  wires:
  io_delay/1 -> cast_gw/1
  cast_gw/1 -> read_write_1_softwareregister3_user_data_in/1
  read_write_1_softwareregister3_user_data_in/1 -> sim_out/1
  out_reg/1 -> reint1/1
  reint1/1 -> io_delay/1
